simulink model "Closed_loop_PI_control_of_DC_DC_Cascode_Buck_Boost_Converter"  (R2019a)
settings: Solver=VariableStepAuto  StartTime=0.0  StopTime=10  RelTol=1e-3
libraries: powerlib x12, powerlib_meascontrol x1, simulink x1
settings Model: Creator=Deepak  LastModifiedBy=Deepak

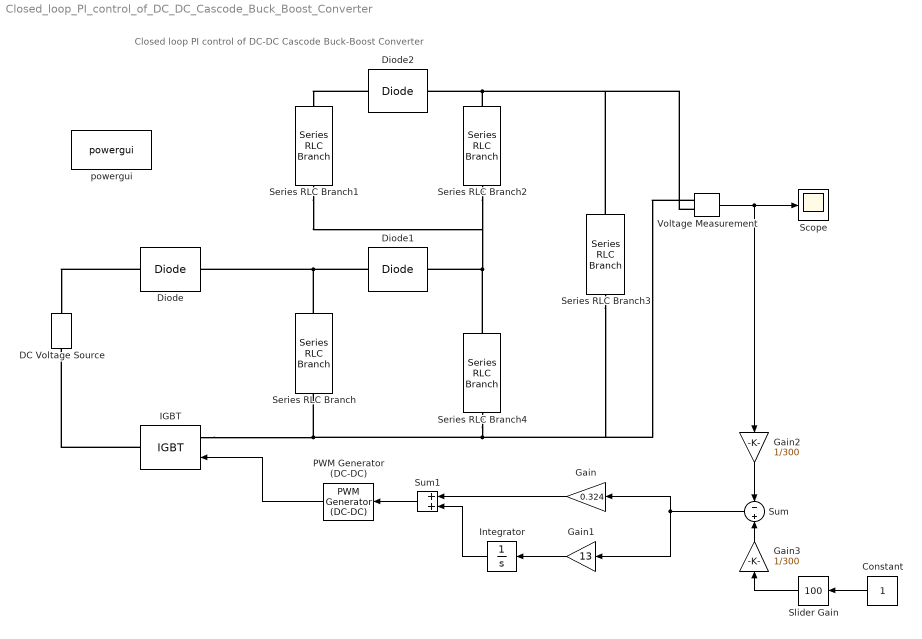
== system Closed_loop_PI_control_of_DC_DC_Cascode_Buck_Boost_Converter ==
  note: Closed loop PI control of DC-DC Cascode Buck-Boost Converter
  Constant : Constant
  DC Voltage Source : powerlib/Electrical Sources/DC Voltage Source  Amplitude=50  Measurements=None
      settings: SourceProductName=Simscape Electrical
  Diode : powerlib/Power Electronics/Diode  Ron=0.001  Lon=0  Vf=0  IC=0  UseSnubber=0  Rs=500  Cs=250e-9  Measurements=off
      settings: SourceProductName=Simscape Electrical
  Diode1 : powerlib/Power Electronics/Diode  Ron=0.001  Lon=0  Vf=0  IC=0  UseSnubber=0  Rs=500  Cs=250e-9  Measurements=off
      settings: SourceProductName=Simscape Electrical
  Diode2 : powerlib/Power Electronics/Diode  Ron=0.001  Lon=0  Vf=0  IC=0  UseSnubber=0  Rs=500  Cs=250e-9  Measurements=off
      settings: SourceProductName=Simscape Electrical
  Gain : Gain  Gain=0.324
  Gain1 : Gain  Gain=13
  Gain2 : Gain  Gain=1/300
  Gain3 : Gain  Gain=1/300
  IGBT : powerlib/Power Electronics/IGBT  Ron=0.001  Lon=0  Vf=0  Tf=1e-6  Tt=2e-6  IC=0  Rs=1e5  Cs=inf  Measurements=off
      settings: SourceProductName=Simscape Electrical
  Integrator : Integrator
  PWM Generator (DC-DC) : powerlib_meascontrol/Pulse & Signal Generators/PWM Generator (DC-DC)  Fsw=10e3  Ts=0
      settings: SourceProductName=Simscape Electrical
  Scope : Scope
  Series RLC Branch : powerlib/Elements/Series RLC Branch  LConnTagsString=__new0  RConnTagsString=__new0  BranchType=L  Resistance=1  Inductance=3e-3  SetiL0=off  InitialCurrent=0  Capacitance=1e-6  Setx0=off  InitialVoltage=0  Measurements=None
      settings: SourceProductName=Simscape Electrical
  Series RLC Branch1 : powerlib/Elements/Series RLC Branch  LConnTagsString=__new0  RConnTagsString=__new0  BranchType=L  Resistance=1  Inductance=16e-3  SetiL0=off  InitialCurrent=0  Capacitance=1e-6  Setx0=off  InitialVoltage=0  Measurements=None
      settings: SourceProductName=Simscape Electrical
  Series RLC Branch2 : powerlib/Elements/Series RLC Branch  LConnTagsString=__new0  RConnTagsString=__new0  BranchType=C  Resistance=1  Inductance=1e-3  SetiL0=off  InitialCurrent=0  Capacitance=100e-6  Setx0=off  InitialVoltage=0  Measurements=None
      settings: SourceProductName=Simscape Electrical
  Series RLC Branch3 : powerlib/Elements/Series RLC Branch  LConnTagsString=__new0  RConnTagsString=__new0  BranchType=R  Resistance=200  Inductance=1e-3  SetiL0=off  InitialCurrent=0  Capacitance=1e-6  Setx0=off  InitialVoltage=0  Measurements=None
      settings: SourceProductName=Simscape Electrical
  Series RLC Branch4 : powerlib/Elements/Series RLC Branch  LConnTagsString=__new0  RConnTagsString=__new0  BranchType=C  Resistance=1  Inductance=1e-3  SetiL0=off  InitialCurrent=0  Capacitance=100e-6  Setx0=off  InitialVoltage=0  Measurements=None
      settings: SourceProductName=Simscape Electrical
  Slider Gain : simulink/Math Operations/Slider Gain  gain=100  low=0  high=250
  Sum : Sum  Inputs=-+
  Sum1 : Sum
  Voltage Measurement : powerlib/Measurements/Voltage Measurement  PhasorSimulation=off  OutputType=Complex  PSBequivalent=0
      settings: SourceProductName=Simscape Electrical
  powergui : powerlib/powergui  Priority=1  SimulationMode=Discrete  SampleTime=1e-6  frequency=60  Iterations=50  frequencyindice=0  Pbase=100e6  ErrMax=1e-4  UnitsV=kV  UnitsW=MW  buscounter=0  FunctionMessages=off  echomessages=off  EnableUseOfTLC=off  CurrentSourceSwitches=off  DisableSnubberDevices=off  DisableRonSwitches=off  DisableVfSwitches=off  DisplayEquations=off  AutomaticDiscreteSolvers=off  SolverType=Tustin/Backward Euler (TBE)  Interpol=off  ExternalGateDelay=off  methode=off  Ts=100  x0status=blocks  SPID=on  SwTol=0  HookPort=off  NonlinearTolerance=0  nMaxIteration=15  ContinueOnMaxIteration=off  RestoreLinks=warning  ResistiveCurrentMeasurement=off  Frange=[0:2:500]  Ylog=off  Xlog=on  ShowGrid=off  save=off  variable=ZData  structure=0  ZoomFFT=off  StartTime=0.0  cycles=1  DisplayStyle=1  fundamental=60  FreqAxis=off  MaxFrequency=1000  frequencyindicesteady=1  RmsSteady=1  display=off
      settings: SourceProductName=Simscape Electrical
  wires:
  Voltage Measurement/1 -> Gain2/1, Scope/1
  Slider Gain/1 -> Gain3/1
  Sum/1 -> Gain/1, Gain1/1
  Gain1/1 -> Integrator/1
  Gain/1 -> Sum1/1
  Integrator/1 -> Sum1/2
  Sum1/1 -> PWM Generator (DC-DC)/1
  PWM Generator (DC-DC)/1 -> IGBT/1
  Constant/1 -> Slider Gain/1
  Gain2/1 -> Sum/1
  Gain3/1 -> Sum/2
  connections:
  Diode1/RConn1 -- Series RLC Branch/RConn1 -- Diode/RConn1
  Diode2/RConn1 -- Series RLC Branch1/RConn1
  Diode/LConn1 -- DC Voltage Source/RConn1
  IGBT/RConn1 -- DC Voltage Source/LConn1
  IGBT/LConn1 -- Series RLC Branch3/LConn1 -- Voltage Measurement/LConn1 -- Series RLC Branch4/LConn1 -- Series RLC Branch/LConn1
  Series RLC Branch2/RConn1 -- Series RLC Branch3/RConn1 -- Voltage Measurement/LConn2 -- Diode2/LConn1
  Series RLC Branch4/RConn1 -- Series RLC Branch2/LConn1 -- Series RLC Branch1/LConn1 -- Diode1/LConn1
